simulink model "fmasse_var2"  (Simulink 4.00)
settings: Solver=ode45  StartTime=0.0  StopTime=10.0  RelTol=1e-3
values from neighbouring files (symbols this model uses):
  a = -1    [fmasse_var_1.m]    (also in fmasse_var_2.m; mehrw_4.m = my_system1.a; mehrw_5.m = my_system1.a)
  D1 = ((2*pi*f1)^2)*m1    (= 394784.176044)    [fmasse_var_1.m]    (also in fmasse_var_2.m)
  D2 = ((2*pi*f2)^2)*m2    (= 39478.4176044)    [fmasse_var_1.m]    (also in fmasse_var_2.m)
  hoehe = 10    [fmasse_var_2.m]
  m1 = 100    [fmasse_var_1.m]    (also in fmasse_var_2.m)
  m2 = 1000    [fmasse_var_1.m]    (also in fmasse_var_2.m)
  r1 = d1*2*sqrt(D1*m1)    [fmasse_var_1.m]    (also in fmasse_var_2.m)
  r21 = d2*2*sqrt(D2*m2)    [fmasse_var_2.m]
  r22 = 3*r21    [fmasse_var_2.m]
  rampe = hoehe/(laenge/V)    (= 111.111111111)    [fmasse_var_2.m]
  Varianz = W/(2*d_t)/V    (= 180)    [fmasse_var_1.m]    (also in fmasse_var_2.m)
settings Model: LastModifiedBy=Administrator  BlockReductionOpt=off

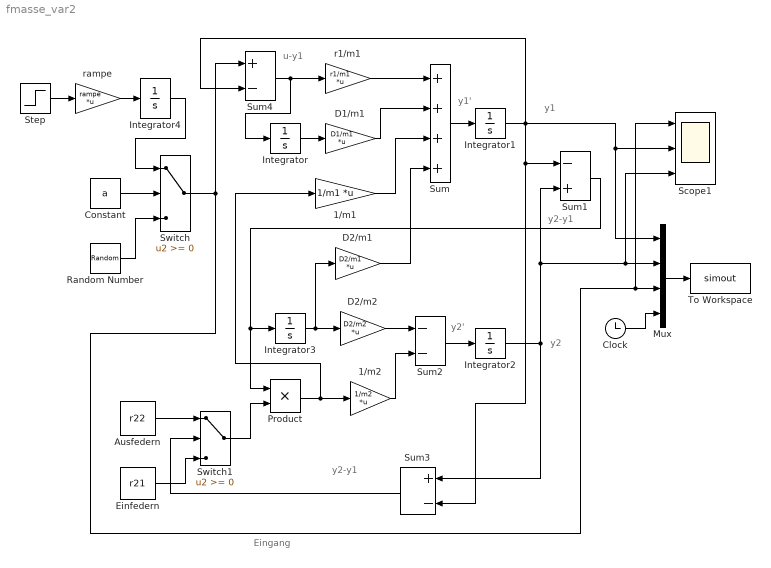
== system fmasse_var2 ==
  note: y1
  note: y1'
  note: y2
  note: y2'
  note: Eingang
  note: u-y1
  note: y2-y1
  note: y2-y1
  1/m1 : Gain  Gain=1/m1  Multiplication=Matrix(K*u)  SaturateOnIntegerOverflow=on
  1/m2 : Gain  Gain=1/m2  Multiplication=Matrix(K*u)  SaturateOnIntegerOverflow=on
  Ausfedern : Constant  Value=r22
  Clock : Clock
      settings: DisplayTime=off  Decimation=10
  Constant : Constant  Value=a
  D1/m1 : Gain  Gain=D1/m1  Multiplication=Matrix(K*u)  SaturateOnIntegerOverflow=on
  D2/m1 : Gain  Gain=D2/m1  Multiplication=Matrix(K*u)  SaturateOnIntegerOverflow=on
  D2/m2 : Gain  Gain=D2/m2  Multiplication=Matrix(K*u)  SaturateOnIntegerOverflow=on
  Einfedern : Constant  Value=r21
  Integrator{,1..3} (4 alike) : Integrator  ExternalReset=none  InitialConditionSource=internal  InitialCondition=0  LimitOutput=off  UpperSaturationLimit=inf  LowerSaturationLimit=-inf  ShowSaturationPort=off  ShowStatePort=off  AbsoluteTolerance=auto
  Integrator4 : Integrator  ExternalReset=none  InitialConditionSource=internal  InitialCondition=0  LimitOutput=on  UpperSaturationLimit=hoehe  LowerSaturationLimit=-inf  ShowSaturationPort=off  ShowStatePort=off  AbsoluteTolerance=auto
  Mux : Mux  Inputs=4
  Product : Product  Inputs=2  Multiplication=Element-wise(.*)  SaturateOnIntegerOverflow=on
  Random Number : RandomNumber  Mean=0  Variance=Varianz  Seed=0  SampleTime=0
  Scope1 : Scope  NumInputPorts=3
      settings: TimeRange=auto  YMin=-200~-30~-10  YMax=200~30~12.5  SaveToWorkspace=off  MaxDataPoints=5000
  Step : Step  Time=0  Before=0  After=1  SampleTime=0
  Sum : Sum  Inputs=++++  SaturateOnIntegerOverflow=on
  Sum1 : Sum  Inputs=-+  SaturateOnIntegerOverflow=on
  Sum2 : Sum  Inputs=--  SaturateOnIntegerOverflow=on
  Sum3 : Sum  Orientation=left  Inputs=+-  SaturateOnIntegerOverflow=on
  Sum4 : Sum  Inputs=+-  SaturateOnIntegerOverflow=on
  Switch : Switch  Threshold=0
  Switch1 : Switch  Threshold=0
  To Workspace : ToWorkspace  VariableName=simout  SampleTime=-1  SaveFormat=Array
  r1/m1 : Gain  Gain=r1/m1  Multiplication=Matrix(K*u)  SaturateOnIntegerOverflow=on
  rampe : Gain  Gain=rampe  Multiplication=Matrix(K*u)  SaturateOnIntegerOverflow=on
  wires:
  Mux/1 -> To Workspace/1
  Integrator1/1 -> Sum4/2, Mux/1, Scope1/2, Sum1/1, Sum3/2
  Integrator2/1 -> Sum1/2, Mux/2, Scope1/3, Sum3/1
  Sum/1 -> Integrator1/1
  r1/m1/1 -> Sum/1
  Sum4/1 -> r1/m1/1, Integrator/1
  Switch/1 -> Sum4/1, Mux/3, Scope1/1
  Integrator/1 -> D1/m1/1
  D1/m1/1 -> Sum/2
  Sum2/1 -> Integrator2/1
  D2/m2/1 -> Sum2/1
  1/m1/1 -> Sum/3
  Sum1/1 -> Product/1, Integrator3/1
  Integrator3/1 -> D2/m2/1, D2/m1/1
  D2/m1/1 -> Sum/4
  Clock/1 -> Mux/4
  Random Number/1 -> Switch/3
  Constant/1 -> Switch/2
  Product/1 -> 1/m2/1, 1/m1/1
  Ausfedern/1 -> Switch1/1
  Einfedern/1 -> Switch1/3
  Switch1/1 -> Product/2
  Sum3/1 -> Switch1/2
  1/m2/1 -> Sum2/2
  Step/1 -> rampe/1
  rampe/1 -> Integrator4/1
  Integrator4/1 -> Switch/1
